simulink model "gm_sampleModel2039_sub"  (R2023a)
settings: Solver=VariableStepAuto  StartTime=0.0  StopTime=10.0  RelTol=1e-3
libraries: simulink x3, hdlsllib x2
settings Model: Creator=user1  LastModifiedBy=user1
settings OptimizationCC: BlockReduction=off  ConditionallyExecuteInputs=off
settings DebuggingCC: InheritedTsInSrcMsg=none

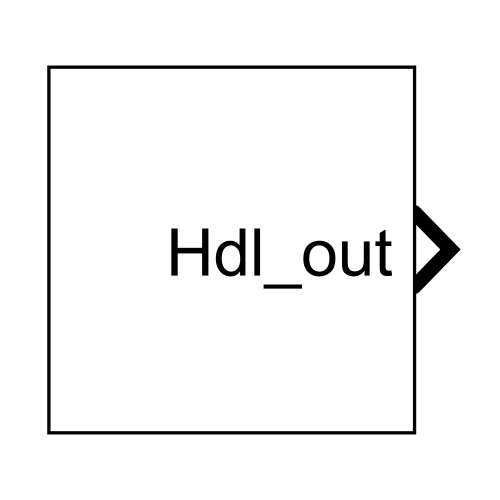
[thumbnail: Simulink's stored preview of the top-level diagram]
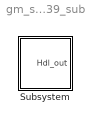
== system gm_sampleModel2039_sub ==
  Subsystem : Subsystem

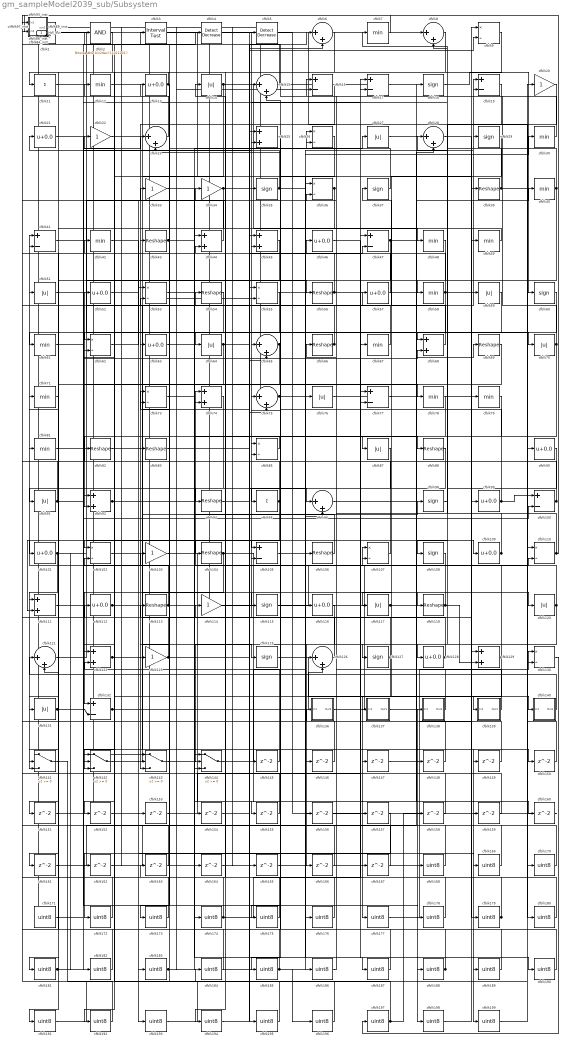
== system gm_sampleModel2039_sub/Subsystem ==
  cfblk1 : hdlsllib/Logic and Bit Operations/Bit Slice  lidx=7  ridx=0
  cfblk{16..17,19,41,47,77,100,105,132} (9 alike) : Sum  Inputs=+-  OutDataTypeStr=uint8
  cfblk{13,21,46,52,57,63,90,99,101,109,112,116,128} (13 alike) : Bias  Bias=0.0  SaturateOnIntegerOverflow=off
  cfblk{9,26,36,53,55,62,73,85,102,107,110,130} (12 alike) : Product  Inputs=*/  OutDataTypeStr=uint8  RndMeth=Zero  SaturateOnIntegerOverflow=on
  cfblk{20,22,33..34,103,114,123} (7 alike) : Gain  OutDataTypeStr=uint8
  cfblk{39,43,54,56,66,69,82..83,88,94,104,106,113,118} (14 alike) : Reshape
  cfblk{18,29,35,37,60,98,108,115,125,127} (10 alike) : Signum
  cfblk10_inst : Subsystem
  cfblk11 : Sum  Inputs=+  OutDataTypeStr=uint8
  cfblk{25,44..45,68,74,92,111,122,129} (9 alike) : Sum  OutDataTypeStr=uint8
  cfblk{14,27,51,59,64,70,76,87,91,117,120,131} (12 alike) : Abs  OutDataTypeStr=uint8  SaturateOnIntegerOverflow=off
  cfblk{7,12,30,40,42,48..49,58,61,67,71,78..79,81} (14 alike) : MinMax  OutDataTypeStr=uint8
  cfblk{6,8,15,23,28,65,75,96,121,126} (10 alike) : Sum  Inputs=|++  OutDataTypeStr=uint8
  cfblk124_inst : Subsystem
  cfblk136 : Subsystem
  cfblk137 : Subsystem
  cfblk138 : Subsystem
  cfblk139 : Subsystem
  cfblk140 : Subsystem
  cfblk{141..144} (4 alike) : Switch  OutDataTypeStr=uint8  SaturateOnIntegerOverflow=off  InputSameDT=off
  cfblk{145..167} (23 alike) : Delay  SampleTime=1
  cfblk{168..199} (32 alike) : DataTypeConversion  OutDataTypeStr=uint8  SaturateOnIntegerOverflow=off  RndMeth=Floor
  cfblk2 : simulink/Logic and Bit Operations/Bitwise Operator  logicop=AND  UseBitMask=on  BitMask=bin2dec('11011001')  BitMaskRealWorld=Stored Integer
      settings: LibrarySourceBlock=|
      | hdlsllib/Logic and Bit
      | Operations/Bitwise
      | Operator
  cfblk3 : hdlsllib/Logic and Bit Operations/Interval Test  IntervalClosedRight=on  uplimit=0.5  IntervalClosedLeft=on  lowlimit=-0.5  OutDataTypeStr=uint8
  cfblk32_inst : Subsystem
  cfblk38_inst : Subsystem
  cfblk4 : simulink/Logic and Bit Operations/Detect Decrease  vinit=0.0  OutDataTypeStr=uint8
      settings: LibrarySourceBlock=|
      | hdlsllib/Logic and Bit
      | Operations/Detect
      | Decrease
  cfblk5 : simulink/Logic and Bit Operations/Detect Decrease  vinit=0.0  OutDataTypeStr=uint8
      settings: LibrarySourceBlock=|
      | hdlsllib/Logic and Bit
      | Operations/Detect
      | Decrease
  cfblk50_inst : Subsystem
  cfblk72_inst : Subsystem
  cfblk80_inst : Subsystem
  cfblk84_inst : Subsystem
  cfblk86_inst : Subsystem
  cfblk89_inst : Subsystem
  cfblk93_inst : Subsystem
  cfblk95 : Sum  Inputs=+  OutDataTypeStr=uint8
  cfblk97_inst : Subsystem
  Hdl_out : Outport  OutDataTypeStr=uint8  SampleTime=1
  wires:
  cfblk1/1 -> cfblk68/1, cfblk56/1
  cfblk10_inst/1(out1) -> cfblk8/1
  cfblk100/1 -> cfblk41/1, cfblk5/1
  cfblk101/1 -> cfblk182/1, cfblk141/3, cfblk109/1, cfblk36/2
  cfblk102/1 -> cfblk118/1
  cfblk103/1 -> cfblk155/1
  cfblk104/1 -> cfblk132/1, cfblk150/1
  cfblk105/1 -> cfblk106/1
  cfblk106/1 -> cfblk74/1
  cfblk107/1 -> cfblk52/1
  cfblk108/1 -> cfblk107/1
  cfblk109/1 -> cfblk54/1, cfblk46/1
  cfblk11/1 -> cfblk143/3
  cfblk110/1 -> cfblk86_inst/2(in2), cfblk28/1
  cfblk111/1 -> cfblk19/1
  cfblk112/1 -> cfblk57/1, cfblk199/1, cfblk144/2, cfblk165/1
  cfblk113/1 -> cfblk44/1, cfblk81/1
  cfblk114/1 -> cfblk177/1
  cfblk115/1 -> cfblk67/1
  cfblk116/1 -> cfblk144/1
  cfblk117/1 -> cfblk69/1, Hdl_out/1
  cfblk118/1 -> cfblk44/2, cfblk129/2
  cfblk12/1 -> cfblk195/1
  cfblk120/1 -> cfblk74/2, cfblk166/1
  cfblk121/1 -> cfblk47/1
  cfblk122/1 -> cfblk98/1, cfblk142/3, cfblk125/1
  cfblk123/1 -> cfblk6/2, cfblk113/1
  cfblk124_inst/1(out1) -> cfblk153/1
  cfblk125/1 -> cfblk140/1(In1)
  cfblk126/1 -> cfblk34/1
  cfblk127/1 -> cfblk124_inst/2(in2), cfblk152/1
  cfblk128/1 -> cfblk65/1, cfblk126/1
  cfblk129/1 -> cfblk85/1, cfblk167/1
  cfblk13/1 -> cfblk173/1, cfblk11/1
  cfblk130/1 -> cfblk197/1
  cfblk131/1 -> cfblk132/2, cfblk110/2
  cfblk132/1 -> cfblk176/1, cfblk126/2
  cfblk136/1(Out1) -> cfblk90/1
  cfblk137/1(Out1) -> cfblk198/1
  cfblk138/1(Out1) -> cfblk36/1
  cfblk139/1(Out1) -> cfblk45/2
  cfblk14/1 -> cfblk142/2, cfblk48/1
  cfblk140/1(Out1) -> cfblk121/1
  cfblk141/1 -> cfblk184/1
  cfblk142/1 -> cfblk49/1
  cfblk143/1 -> cfblk103/1
  cfblk144/1 -> cfblk29/1
  cfblk145/1 -> cfblk122/2
  cfblk146/1 -> cfblk84_inst/1(in1)
  cfblk147/1 -> cfblk129/1
  cfblk148/1 -> cfblk10_inst/2(in2)
  cfblk149/1 -> cfblk15/2
  cfblk15/1 -> cfblk84_inst/2(in2)
  cfblk150/1 -> cfblk110/1
  cfblk151/1 -> cfblk68/2
  cfblk152/1 -> cfblk193/1
  cfblk153/1 -> cfblk17/2
  cfblk154/1 -> cfblk47/2
  cfblk155/1 -> cfblk102/2
  cfblk156/1 -> cfblk77/1
  cfblk157/1 -> cfblk172/1
  cfblk158/1 -> cfblk97_inst/2(in2)
  cfblk159/1 -> cfblk121/2
  cfblk16/1 -> cfblk63/1
  cfblk160/1 -> cfblk1/1
  cfblk161/1 -> cfblk28/2
  cfblk162/1 -> cfblk55/1
  cfblk163/1 -> cfblk93_inst/1(in1)
  cfblk164/1 -> cfblk45/1
  cfblk165/1 -> cfblk96/2
  cfblk166/1 -> cfblk75/1
  cfblk167/1 -> cfblk89_inst/2(in2)
  cfblk168/1 -> cfblk66/1
  cfblk169/1 -> cfblk80_inst/1(in1)
  cfblk17/1 -> cfblk138/1(In1)
  cfblk170/1 -> cfblk80_inst/2(in2)
  cfblk171/1 -> cfblk100/2
  cfblk172/1 -> cfblk38_inst/1(in1)
  cfblk173/1 -> cfblk38_inst/2(in2)
  cfblk174/1 -> cfblk77/2, cfblk65/2, cfblk32_inst/2(in2)
  cfblk175/1 -> cfblk73/1
  cfblk176/1 -> cfblk73/2
  cfblk177/1 -> cfblk99/1
  cfblk178/1 -> cfblk114/1
  cfblk179/1 -> cfblk51/1, cfblk41/2, cfblk62/2, cfblk136/1(In1)
  cfblk18/1 -> cfblk60/1
  cfblk180/1 -> cfblk22/1
  cfblk181/1 -> cfblk25/2, cfblk17/1, cfblk107/2
  cfblk182/1 -> cfblk71/1
  cfblk183/1 -> cfblk105/2, cfblk163/1
  cfblk184/1 -> cfblk42/1
  cfblk185/1 -> cfblk76/1, cfblk196/1, cfblk53/2
  cfblk186/1 -> cfblk26/1
  cfblk187/1 -> cfblk26/2
  cfblk188/1 -> cfblk50_inst/2(in2), cfblk85/2
  cfblk189/1 -> cfblk33/1
  cfblk19/1 -> cfblk128/1
  cfblk190/1 -> cfblk2/1
  cfblk191/1 -> cfblk20/1
  cfblk192/1 -> cfblk97_inst/1(in1)
  cfblk193/1 -> cfblk9/1
  cfblk194/1 -> cfblk9/2
  cfblk195/1 -> cfblk112/1
  cfblk196/1 -> cfblk12/1
  cfblk197/1 -> cfblk13/1, cfblk158/1
  cfblk198/1 -> cfblk130/1
  cfblk199/1 -> cfblk130/2
  cfblk2/1 -> cfblk191/1
  cfblk20/1 -> cfblk58/1
  cfblk21/1 -> cfblk178/1
  cfblk22/1 -> cfblk179/1
  cfblk23/1 -> cfblk93_inst/2(in2)
  cfblk25/1 -> cfblk175/1
  cfblk26/1 -> cfblk185/1
  cfblk27/1 -> cfblk159/1
  cfblk28/1 -> cfblk39/1
  cfblk29/1 -> cfblk127/1
  cfblk3/1 -> cfblk156/1
  cfblk30/1 -> cfblk32_inst/1(in1)
  cfblk32_inst/1(out1) -> cfblk154/1
  cfblk33/1 -> cfblk188/1
  cfblk34/1 -> cfblk116/1, cfblk151/1
  cfblk35/1 -> cfblk70/1, cfblk21/1
  cfblk36/1 -> cfblk194/1, cfblk62/1
  cfblk37/1 -> cfblk89_inst/1(in1)
  cfblk38_inst/1(out1) -> cfblk171/1
  cfblk39/1 -> cfblk180/1, cfblk15/1
  cfblk4/1 -> cfblk157/1
  cfblk40/1 -> cfblk101/1, cfblk7/1
  cfblk41/1 -> cfblk4/1
  cfblk42/1 -> cfblk183/1
  cfblk43/1 -> cfblk27/1, cfblk160/1
  cfblk44/1 -> cfblk10_inst/1(in1)
  cfblk45/1 -> cfblk131/1
  cfblk46/1 -> cfblk189/1
  cfblk47/1 -> cfblk111/1, cfblk40/1
  cfblk48/1 -> cfblk94/1
  cfblk49/1 -> cfblk43/1
  cfblk5/1 -> cfblk170/1
  cfblk50_inst/1(out1) -> cfblk143/1
  cfblk51/1 -> cfblk78/1
  cfblk52/1 -> cfblk169/1
  cfblk53/1 -> cfblk88/1
  cfblk54/1 -> cfblk141/2
  cfblk55/1 -> cfblk102/1
  cfblk56/1 -> cfblk86_inst/1(in1), cfblk124_inst/1(in1)
  cfblk57/1 -> cfblk16/1
  cfblk58/1 -> cfblk87/1, cfblk25/1, cfblk61/1
  cfblk59/1 -> cfblk122/1
  cfblk6/1 -> cfblk104/1
  cfblk60/1 -> cfblk64/1
  cfblk61/1 -> cfblk23/1
  cfblk62/1 -> cfblk35/1
  cfblk63/1 -> cfblk115/1
  cfblk64/1 -> cfblk190/1, cfblk144/3
  cfblk65/1 -> cfblk142/1, cfblk105/1, cfblk162/1
  cfblk66/1 -> cfblk50_inst/1(in1), cfblk3/1
  cfblk67/1 -> cfblk53/1
  cfblk68/1 -> cfblk37/1
  cfblk69/1 -> cfblk91/1
  cfblk7/1 -> cfblk72_inst/1(in1)
  cfblk70/1 -> cfblk19/2, cfblk117/1
  cfblk71/1 -> cfblk181/1
  cfblk72_inst/1(out1) -> cfblk164/1
  cfblk73/1 -> cfblk174/1
  cfblk74/1 -> cfblk161/1
  cfblk75/1 -> cfblk187/1, cfblk30/1
  cfblk76/1 -> cfblk120/1
  cfblk77/1 -> cfblk137/1(In1)
  cfblk78/1 -> cfblk92/2
  cfblk79/1 -> cfblk82/1
  cfblk8/1 -> cfblk92/1
  cfblk80_inst/1(out1) -> cfblk168/1
  cfblk81/1 -> cfblk146/1
  cfblk82/1 -> cfblk6/1
  cfblk83/1 -> cfblk96/1
  cfblk84_inst/1(out1) -> cfblk16/2, cfblk79/1
  cfblk85/1 -> cfblk83/1
  cfblk86_inst/1(out1) -> cfblk186/1, cfblk18/1
  cfblk87/1 -> cfblk95/1
  cfblk88/1 -> cfblk123/1
  cfblk89_inst/1(out1) -> cfblk59/1
  cfblk9/1 -> cfblk192/1
  cfblk90/1 -> cfblk108/1
  cfblk91/1 -> cfblk72_inst/2(in2), cfblk143/2
  cfblk92/1 -> cfblk149/1, cfblk148/1, cfblk147/1
  cfblk93_inst/1(out1) -> cfblk141/1
  cfblk94/1 -> cfblk75/2
  cfblk95/1 -> cfblk14/1, cfblk111/2
  cfblk96/1 -> cfblk139/1(In1)
  cfblk97_inst/1(out1) -> cfblk55/2, cfblk145/1
  cfblk98/1 -> cfblk8/2
  cfblk99/1 -> cfblk23/2, cfblk100/1

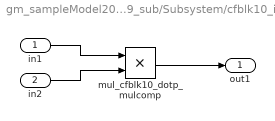
== system gm_sampleModel2039_sub/Subsystem/cfblk10_inst ==
  in1 : Inport  OutDataTypeStr=uint8  SampleTime=1
  in2 : Inport  Port=2  OutDataTypeStr=uint8  SampleTime=1
  mul_cfblk10_dotp_mulcomp : Product  Inputs=**  OutDataTypeStr=uint8  SampleTime=1
  out1 : Outport  OutDataTypeStr=uint8  SampleTime=1
  wires:
  in1/1 -> mul_cfblk10_dotp_mulcomp/1
  in2/1 -> mul_cfblk10_dotp_mulcomp/2
  mul_cfblk10_dotp_mulcomp/1 -> out1/1

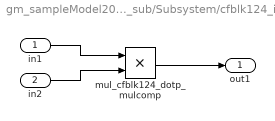
== system gm_sampleModel2039_sub/Subsystem/cfblk124_inst ==
  in1 : Inport  OutDataTypeStr=uint8  SampleTime=1
  in2 : Inport  Port=2  OutDataTypeStr=uint8  SampleTime=1
  mul_cfblk124_dotp_mulcomp : Product  Inputs=**  OutDataTypeStr=uint8  SampleTime=1
  out1 : Outport  OutDataTypeStr=uint8  SampleTime=1
  wires:
  in1/1 -> mul_cfblk124_dotp_mulcomp/1
  in2/1 -> mul_cfblk124_dotp_mulcomp/2
  mul_cfblk124_dotp_mulcomp/1 -> out1/1

== system gm_sampleModel2039_sub/Subsystem/cfblk136 ==
  In1 : Inport  OutDataTypeStr=uint8  PortDimensions=1  SampleTime=1
  Out1 : Outport  SampleTime=1
  wires:
  In1/1 -> Out1/1

== system gm_sampleModel2039_sub/Subsystem/cfblk137 ==
  In1 : Inport  OutDataTypeStr=uint8  PortDimensions=1  SampleTime=1
  Out1 : Outport  SampleTime=1
  wires:
  In1/1 -> Out1/1

== system gm_sampleModel2039_sub/Subsystem/cfblk138 ==
  In1 : Inport  OutDataTypeStr=uint8  PortDimensions=1  SampleTime=1
  Out1 : Outport  SampleTime=1
  wires:
  In1/1 -> Out1/1

== system gm_sampleModel2039_sub/Subsystem/cfblk139 ==
  In1 : Inport  OutDataTypeStr=uint8  PortDimensions=1  SampleTime=1
  Out1 : Outport  SampleTime=1
  wires:
  In1/1 -> Out1/1

== system gm_sampleModel2039_sub/Subsystem/cfblk140 ==
  In1 : Inport  OutDataTypeStr=uint8  PortDimensions=1  SampleTime=1
  Out1 : Outport  SampleTime=1
  wires:
  In1/1 -> Out1/1

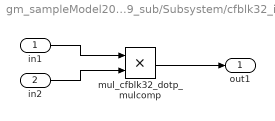
== system gm_sampleModel2039_sub/Subsystem/cfblk32_inst ==
  in1 : Inport  OutDataTypeStr=uint8  SampleTime=1
  in2 : Inport  Port=2  OutDataTypeStr=uint8  SampleTime=1
  mul_cfblk32_dotp_mulcomp : Product  Inputs=**  OutDataTypeStr=uint8  SampleTime=1
  out1 : Outport  OutDataTypeStr=uint8  SampleTime=1
  wires:
  in1/1 -> mul_cfblk32_dotp_mulcomp/1
  in2/1 -> mul_cfblk32_dotp_mulcomp/2
  mul_cfblk32_dotp_mulcomp/1 -> out1/1

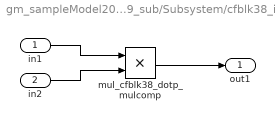
== system gm_sampleModel2039_sub/Subsystem/cfblk38_inst ==
  in1 : Inport  OutDataTypeStr=uint8  SampleTime=1
  in2 : Inport  Port=2  OutDataTypeStr=uint8  SampleTime=1
  mul_cfblk38_dotp_mulcomp : Product  Inputs=**  OutDataTypeStr=uint8  SampleTime=1
  out1 : Outport  OutDataTypeStr=uint8  SampleTime=1
  wires:
  in1/1 -> mul_cfblk38_dotp_mulcomp/1
  in2/1 -> mul_cfblk38_dotp_mulcomp/2
  mul_cfblk38_dotp_mulcomp/1 -> out1/1

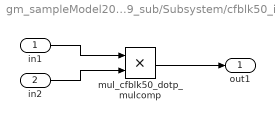
== system gm_sampleModel2039_sub/Subsystem/cfblk50_inst ==
  in1 : Inport  OutDataTypeStr=uint8  SampleTime=1
  in2 : Inport  Port=2  OutDataTypeStr=uint8  SampleTime=1
  mul_cfblk50_dotp_mulcomp : Product  Inputs=**  OutDataTypeStr=uint8  SampleTime=1
  out1 : Outport  OutDataTypeStr=uint8  SampleTime=1
  wires:
  in1/1 -> mul_cfblk50_dotp_mulcomp/1
  in2/1 -> mul_cfblk50_dotp_mulcomp/2
  mul_cfblk50_dotp_mulcomp/1 -> out1/1

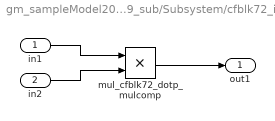
== system gm_sampleModel2039_sub/Subsystem/cfblk72_inst ==
  in1 : Inport  OutDataTypeStr=uint8  SampleTime=1
  in2 : Inport  Port=2  OutDataTypeStr=uint8  SampleTime=1
  mul_cfblk72_dotp_mulcomp : Product  Inputs=**  OutDataTypeStr=uint8  SampleTime=1
  out1 : Outport  OutDataTypeStr=uint8  SampleTime=1
  wires:
  in1/1 -> mul_cfblk72_dotp_mulcomp/1
  in2/1 -> mul_cfblk72_dotp_mulcomp/2
  mul_cfblk72_dotp_mulcomp/1 -> out1/1

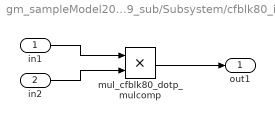
== system gm_sampleModel2039_sub/Subsystem/cfblk80_inst ==
  in1 : Inport  OutDataTypeStr=uint8  SampleTime=1
  in2 : Inport  Port=2  OutDataTypeStr=uint8  SampleTime=1
  mul_cfblk80_dotp_mulcomp : Product  Inputs=**  OutDataTypeStr=uint8  SampleTime=1
  out1 : Outport  OutDataTypeStr=uint8  SampleTime=1
  wires:
  in1/1 -> mul_cfblk80_dotp_mulcomp/1
  in2/1 -> mul_cfblk80_dotp_mulcomp/2
  mul_cfblk80_dotp_mulcomp/1 -> out1/1

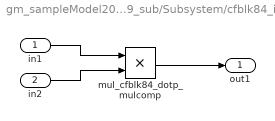
== system gm_sampleModel2039_sub/Subsystem/cfblk84_inst ==
  in1 : Inport  OutDataTypeStr=uint8  SampleTime=1
  in2 : Inport  Port=2  OutDataTypeStr=uint8  SampleTime=1
  mul_cfblk84_dotp_mulcomp : Product  Inputs=**  OutDataTypeStr=uint8  SampleTime=1
  out1 : Outport  OutDataTypeStr=uint8  SampleTime=1
  wires:
  in1/1 -> mul_cfblk84_dotp_mulcomp/1
  in2/1 -> mul_cfblk84_dotp_mulcomp/2
  mul_cfblk84_dotp_mulcomp/1 -> out1/1

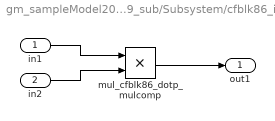
== system gm_sampleModel2039_sub/Subsystem/cfblk86_inst ==
  in1 : Inport  OutDataTypeStr=uint8  SampleTime=1
  in2 : Inport  Port=2  OutDataTypeStr=uint8  SampleTime=1
  mul_cfblk86_dotp_mulcomp : Product  Inputs=**  OutDataTypeStr=uint8  SampleTime=1
  out1 : Outport  OutDataTypeStr=uint8  SampleTime=1
  wires:
  in1/1 -> mul_cfblk86_dotp_mulcomp/1
  in2/1 -> mul_cfblk86_dotp_mulcomp/2
  mul_cfblk86_dotp_mulcomp/1 -> out1/1

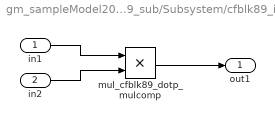
== system gm_sampleModel2039_sub/Subsystem/cfblk89_inst ==
  in1 : Inport  OutDataTypeStr=uint8  SampleTime=1
  in2 : Inport  Port=2  OutDataTypeStr=uint8  SampleTime=1
  mul_cfblk89_dotp_mulcomp : Product  Inputs=**  OutDataTypeStr=uint8  SampleTime=1
  out1 : Outport  OutDataTypeStr=uint8  SampleTime=1
  wires:
  in1/1 -> mul_cfblk89_dotp_mulcomp/1
  in2/1 -> mul_cfblk89_dotp_mulcomp/2
  mul_cfblk89_dotp_mulcomp/1 -> out1/1

== system gm_sampleModel2039_sub/Subsystem/cfblk93_inst ==
  in1 : Inport  OutDataTypeStr=uint8  SampleTime=1
  in2 : Inport  Port=2  OutDataTypeStr=uint8  SampleTime=1
  mul_cfblk93_dotp_mulcomp : Product  Inputs=**  OutDataTypeStr=uint8  SampleTime=1
  out1 : Outport  OutDataTypeStr=uint8  SampleTime=1
  wires:
  in1/1 -> mul_cfblk93_dotp_mulcomp/1
  in2/1 -> mul_cfblk93_dotp_mulcomp/2
  mul_cfblk93_dotp_mulcomp/1 -> out1/1

== system gm_sampleModel2039_sub/Subsystem/cfblk97_inst ==
  in1 : Inport  OutDataTypeStr=uint8  SampleTime=1
  in2 : Inport  Port=2  OutDataTypeStr=uint8  SampleTime=1
  mul_cfblk97_dotp_mulcomp : Product  Inputs=**  OutDataTypeStr=uint8  SampleTime=1
  out1 : Outport  OutDataTypeStr=uint8  SampleTime=1
  wires:
  in1/1 -> mul_cfblk97_dotp_mulcomp/1
  in2/1 -> mul_cfblk97_dotp_mulcomp/2
  mul_cfblk97_dotp_mulcomp/1 -> out1/1
